simulink model "lab754_rtlsdr_qpsk_coarse_synch"  (R2018b)
settings: Solver=VariableStepAuto  StartTime=0.0  StopTime=inf  RelTol=1e-3
PreLoadFcn:
  | Hd1 = dsp.FIRDecimator (5);
  | Hd2 = dsp.FIRDecimator (6);
undefined symbols (not defined in the file): designMultirateFIR
libraries: dspmlti4 x2, sdrrlib x1, commfilt2 x1, dspspect3 x1, dspstat3 x1, commrflib2 x1
settings Model: Creator=Григорий Фокин  LastModifiedBy=Григорий Фокин

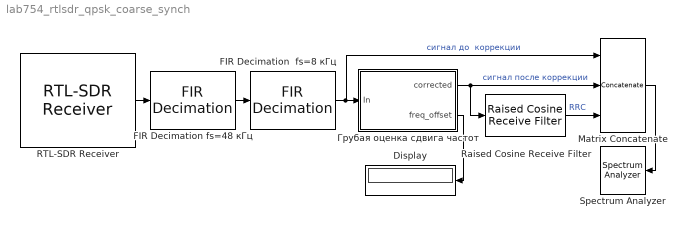
== system lab754_rtlsdr_qpsk_coarse_synch ==
  Display : Display
  FIR Decimation  fs=8 кГц : dspmlti4/FIR Decimation  FilterSource=Filter object  h=designMultirateFIR(1,2)  D=2  filtStruct=Direct form  FilterObject=Hd2  InputProcessing=Columns as channels (frame based)  framing=Allow multirate processing  inputOffset=0  outputBufInitCond=0  roundingMode=Floor  overflowMode=off  firstCoeffDataTypeStr=Inherit: Same word length as input  firstCoeffMin=[]  firstCoeffMax=[]  firstCoeffLastDataTypeStr=Inherit: Same word length as input  outputDataTypeStr=Inherit: Same as accumulator  outputMin=[]  outputMax=[]  outputLastDataTypeStr=Inherit: Same as accumulator
  FIR Decimation fs=48 кГц : dspmlti4/FIR Decimation  FilterSource=Filter object  h=designMultirateFIR(1,2)  D=2  filtStruct=Direct form  FilterObject=Hd1  InputProcessing=Columns as channels (frame based)  framing=Allow multirate processing  inputOffset=0  outputBufInitCond=0  roundingMode=Floor  overflowMode=off  firstCoeffDataTypeStr=Inherit: Same word length as input  firstCoeffMin=[]  firstCoeffMax=[]  firstCoeffLastDataTypeStr=Inherit: Same word length as input  outputDataTypeStr=Inherit: Same as accumulator  outputMin=[]  outputMax=[]  outputLastDataTypeStr=Inherit: Same as accumulator
  Matrix Concatenate : Concatenate  NumInputs=3  Mode=Multidimensional array  ConcatenateDimension=2
  RTL-SDR Receiver : sdrrlib/RTL-SDR Receiver  IPAddress=0  CenterFrequencySource=Dialog  CenterFrequency=1200e6+500  GainSource=AGC  Gain=40  ADCRate=240e3  FrequencyCorrection=47  LostSamplesOutputPort=off  LatencyOutputPort=off  OutputDataType=double  FrameLength=4096  EnableBurstMode=off  NumFramesInBurst=20  sobjType=sdrr.internal.SDRRTLReceiverSL  dataUDPPort=-1  ctrlUDPPort=-1  subDeviceList=nosubdev  sdrBlockType=SDRBlockTypeSLT.SDRRxBlock  requester=UNUSED_BY_SFCN  sdrExecutionMode=SDRExecutionModeSLT.ExecModeHW  BypassUserLogic=off  DecimatorSelect=DDC decimator  SourceSelect=RF data  SineAmplitude=16000  EnableInternalClock=off  BypassIQBalance=off  IFBandwidth=40e6  ADCRateSource=Dialog  IntermediateFrequency=0  DecimationFactorSource=Dialog  DecimationFactor=512  RFFrequencyIsTunable=logical(0)  SampleTime=(4096)/(240e3)  IFBandwidthSource=Dialog  SineFrequency=30000  BypassDCBlockingFilter=off  IntermediateFrequencySource=Dialog  IQBalanceCoefficients=64  SkipAllHardwareResetAndInitialization=off  EnableIQCalibrationTable=on  CacheIQCalibrationTable=off  EnableOffsetTuning=off  EnableRTLAGC=off  EnableTestMode=off  EnableTunerAGC=on  FrequencyCorrectionSource=Dialog  NumMLBuffers=128  NumUSBBuffers=16  RTLCrystalFrequency=28800000  TunerCrystalFrequency=28800000
      settings: SourceProductName=Communications System Toolbox Support Package for RTL-SDR Radio  SourceProductBaseCode=RTLSDR
  Raised Cosine Receive Filter : commfilt2/Raised Cosine Receive Filter  filtType=Square root  R=0.5  filtSpan=12  N=8  downFactor=1  downOffset=0  filterGain=1  InputProcessing=Columns as channels (frame based)  RateOptions=Allow multirate processing  framing=Mute  checkCoeff=off  variableName=rcRxFilt  currentFiltSpan=12  D=(12)/2  inputOffset=0  sampMode=Mute  saveAsFlag=0  rateMode=Downsampling  checkGain=Normalized  launchFVT=on  roundingMode=Floor  overflowMode=off  coeffDataTypeStr=Inherit: Same word length as input  coeffMin=[]  coeffMax=[]  coeffLastDataTypeStr=Inherit: Same word length as input  accumDataTypeStr=Inherit: Same as product output  accumLastDataTypeStr=Inherit: Same as product output  outputDataTypeStr=Inherit: Same as accumulator  outputMin=[]  outputMax=[]  outputLastDataTypeStr=Inherit: Same as accumulator
  Spectrum Analyzer : SpectrumAnalyzer
  Грубая оценка сдвига частот : Subsystem  mask{frame_size=4096}
      mask prompts: frame_size "Размер кадра"
  wires:
  Matrix Concatenate/1 -> Spectrum Analyzer/1
  RTL-SDR Receiver/1 -> FIR Decimation fs=48 кГц/1
  FIR Decimation fs=48 кГц/1 -> FIR Decimation  fs=8 кГц/1
  FIR Decimation  fs=8 кГц/1 -> Matrix Concatenate/1, Грубая оценка сдвига частот/1(In)  "сигнал до  коррекции"
  Грубая оценка сдвига частот/2(freq_offset) -> Display/1
  Грубая оценка сдвига частот/1(corrected) -> Matrix Concatenate/2, Raised Cosine Receive Filter/1  "сигнал после коррекции"
  Raised Cosine Receive Filter/1 -> Matrix Concatenate/3  "RRC"

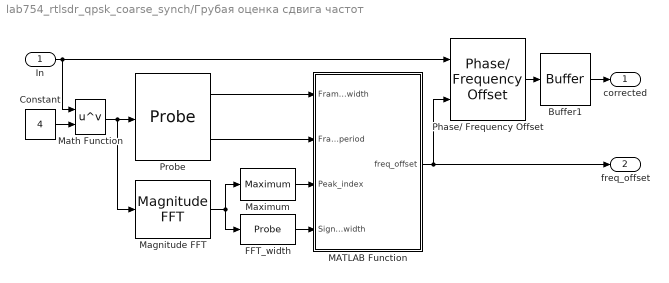
== system lab754_rtlsdr_qpsk_coarse_synch/Грубая оценка сдвига частот ==
  In : Inport
  Buffer1 : Buffer  N=frame_size  OutputFrames=off
  Constant : Constant  Value=4
  FFT_width : Probe  ProbeSampleTime=off  ProbeComplexSignal=off
  MATLAB Function : MATLAB Function  TreatAsAtomicUnit=on
  Magnitude FFT : dspspect3/Magnitude FFT  mag_or_magsq=Magnitude squared  FFTImplementation=Auto  fftLenInherit=on  fftsize=256  WrapInput=on
      settings: SourceProductName=DSP System Toolbox  SourceProductBaseCode=DS
  Math Function : Math  Operator=pow  SaturateOnIntegerOverflow=on
  Maximum : dspstat3/Maximum  operation=maximum  fcn=Index  indexBase=One  operateOver=Each column  Dimension=1  InputProcessing=Columns as channels (frame based)  reset=None  roiEnable=off  roiType=Rectangles  roiPortion=Entire ROI  roiOutput=Individual statistics for each ROI  roiFlag=off  roundingMode=Floor  overflowMode=off  accumDataTypeStr=Inherit: Same as product output  accumLastDataTypeStr=Inherit: Same as product output
  Phase/ Frequency Offset : commrflib2/Phase// Frequency Offset  phaseOffset=0  freqPort=on  freqOffset=0
      settings: SourceProductName=Communications System Toolbox
  Probe : Probe  ProbeComplexSignal=off
  corrected : Outport
  freq_offset : Outport  Port=2
  wires:
  Probe/1 -> MATLAB Function/1(Frame_width)
  Maximum/1 -> MATLAB Function/3(Peak_index)
  FFT_width/1 -> MATLAB Function/4(Signal_width)
  MATLAB Function/1(freq_offset) -> freq_offset/1, Phase/ Frequency Offset/2
  Math Function/1 -> Magnitude FFT/1, Probe/1
  In/1 -> Math Function/1, Phase/ Frequency Offset/1
  Probe/2 -> MATLAB Function/2(Frame_period)
  Constant/1 -> Math Function/2
  Magnitude FFT/1 -> Maximum/1, FFT_width/1
  Buffer1/1 -> corrected/1
  Phase/ Frequency Offset/1 -> Buffer1/1

== matlab function lab754_rtlsdr_qpsk_coarse_synch/Грубая оценка сдвига частот/MATLAB Function ==
  data: Frame_width input; freq_offset output; Frame_period input; Peak_index input; Signal_width input
function freq_offset = fcn(Frame_width,Frame_period,...
                            Peak_index,Signal_width)
% Оценка требуемого индекса сдвига
if Peak_index > Signal_width/2
    offset = (Signal_width+1)-Peak_index;
else
    offset = 1-Peak_index;
end
% оценка периода дискретизации
Ts = Frame_period(1)/Frame_width;
% БПФ разрешение по частоте // fft bin
freq_resolution = 1/(Ts*Signal_width);
% оценка частотного сдвига
freq_offset = offset*freq_resolution/4;
